simulink model "DOF_2"  (R2019b)
settings: Solver=VariableStepAuto  StartTime=0.0  StopTime=10.0  RelTol=1e-3
values from neighbouring files (symbols this model uses):
  c_2 = 7    [DOF_1.mat]    (also in DOF_2.mat)
  k_1 = 2200    [DOF_1.mat]    (also in DOF_2.mat)
  k_2 = 405    [DOF_1.mat]    (also in DOF_2.mat)
  m_1 = 1.5    [DOF_1.mat]    (also in DOF_2.mat)
  m_2 = 6.4    [DOF_2.mat]
settings Model: Creator=MASAHIRO  LastModifiedBy=MASAHIRO

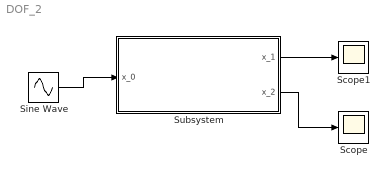
== system DOF_2 ==
  Scope : Scope
  Scope1 : Scope
  Sine Wave : Sin  Amplitude=0.02  SampleTime=0
  Subsystem : Subsystem
  wires:
  Sine Wave/1 -> Subsystem/1(x_0)
  Subsystem/2(x_2) -> Scope/1
  Subsystem/1(x_1) -> Scope1/1

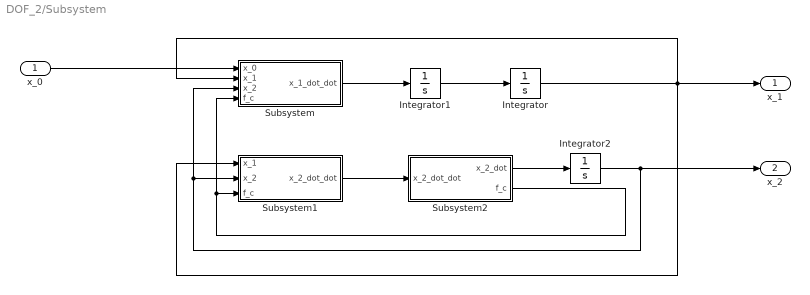
== system DOF_2/Subsystem ==
  x_0 : Inport
  Integrator : Integrator
  Integrator1 : Integrator
  Integrator2 : Integrator
  Subsystem : Subsystem
  Subsystem1 : Subsystem
  Subsystem2 : Subsystem
  x_1 : Outport
  x_2 : Outport  Port=2
  wires:
  Subsystem2/2(f_c) -> Subsystem/4(f_c), Subsystem1/3(f_c)
  Integrator2/1 -> x_2/1, Subsystem1/2(x_2), Subsystem/3(x_2)
  Subsystem1/1(x_2_dot_dot) -> Subsystem2/1(x_2_dot_dot)
  Integrator/1 -> x_1/1, Subsystem/2(x_1), Subsystem1/1(x_1)
  Subsystem/1(x_1_dot_dot) -> Integrator1/1
  Subsystem2/1(x_2_dot) -> Integrator2/1
  Integrator1/1 -> Integrator/1
  x_0/1 -> Subsystem/1(x_0)

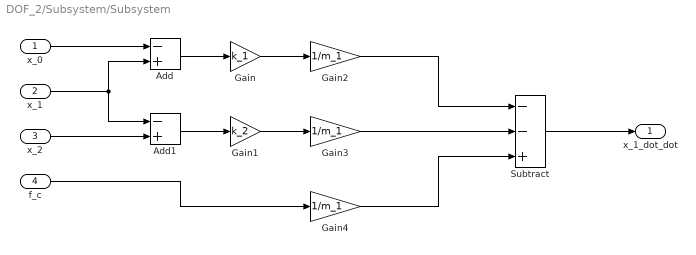
== system DOF_2/Subsystem/Subsystem ==
  x_0 : Inport
  x_1 : Inport  Port=2
  x_2 : Inport  Port=3
  f_c : Inport  Port=4
  Add : Sum  Inputs=-+
  Add1 : Sum  Inputs=-+
  Gain : Gain  Gain=k_1
  Gain1 : Gain  Gain=k_2
  Gain2 : Gain  Gain=1/m_1
  Gain3 : Gain  Gain=1/m_1
  Gain4 : Gain  Gain=1/m_1
  Subtract : Sum  Inputs=--+
  x_1_dot_dot : Outport
  wires:
  x_1/1 -> Add1/1, Add/2
  x_0/1 -> Add/1
  Add/1 -> Gain/1
  Gain/1 -> Gain2/1
  x_2/1 -> Add1/2
  Add1/1 -> Gain1/1
  Gain1/1 -> Gain3/1
  f_c/1 -> Gain4/1
  Gain3/1 -> Subtract/2
  Gain2/1 -> Subtract/1
  Gain4/1 -> Subtract/3
  Subtract/1 -> x_1_dot_dot/1

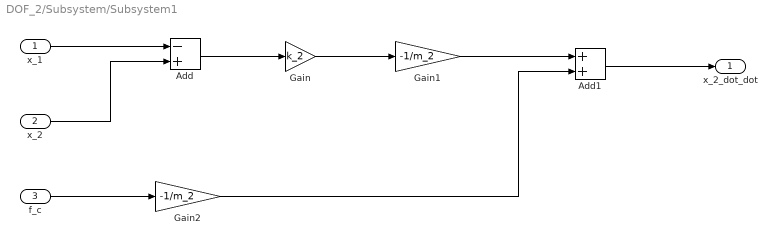
== system DOF_2/Subsystem/Subsystem1 ==
  x_1 : Inport
  x_2 : Inport  Port=2
  f_c : Inport  Port=3
  Add : Sum  Inputs=-+
  Add1 : Sum
  Gain : Gain  Gain=k_2
  Gain1 : Gain  Gain=-1/m_2
  Gain2 : Gain  Gain=-1/m_2
  x_2_dot_dot : Outport
  wires:
  x_1/1 -> Add/1
  x_2/1 -> Add/2
  Add/1 -> Gain/1
  f_c/1 -> Gain2/1
  Gain/1 -> Gain1/1
  Gain1/1 -> Add1/1
  Gain2/1 -> Add1/2
  Add1/1 -> x_2_dot_dot/1

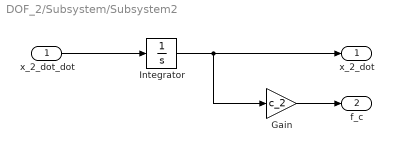
== system DOF_2/Subsystem/Subsystem2 ==
  x_2_dot_dot : Inport
  Gain : Gain  Gain=c_2
  Integrator : Integrator
  x_2_dot : Outport
  f_c : Outport  Port=2
  wires:
  x_2_dot_dot/1 -> Integrator/1
  Integrator/1 -> x_2_dot/1, Gain/1
  Gain/1 -> f_c/1
